simulink model "NCAP_AEBS_Test_T3_CCR_s_cs"  (Simulink 7.6)
settings: Solver=ode5  SolverMode=SingleTasking  StartTime=0.0  StopTime=inf  FixedStep=1/100  RelTol=1e-3
PreLoadFcn:
  | check_NUTS_defined;
  | 
  | assignin('base',['model_closed_' bdroot],false);addpath('../includes_AEBS');
InitFcn:
  | PreScanExperimentInitFcn(bdroot)
StopFcn:
  | PreScanExperimentStopFcn(bdroot)
undefined symbols (not defined in the file): DiscIntNeverNeededParam, x_ini_VRML, y_ini_VRML, z_ini_VRML
libraries: simulink x24, PreScanSimulinkLibrary x10, simulink_extras x7, PreScanUsefulBlocks x5, simulink_need_slupdate x1
(part 4 of 5)

== system NCAP_AEBS_Test_T3_CCR_s_cs/Audi_A8_1/PathFollower_1/CTRL REFERENCES ==
  note: REFERENCE POSITION BASED POSITION CTRL
  Pos x,y,Y [m,m,rad] : Inport
  Position Preview Distance [m] : Inport  Port=2
  TrajOffset [m,m,rad] : Inport  Port=3
  ActorOffset_Left(+) / Right(-)_[m] : Inport  Port=4
  Calculate Preview Point (pvp) by extrapolating current Vehicle Position (p0) with Preview Distance and Vehicle Orientation : Subsystem
  Find Reference Point (pref)  on Trajectory closest  to PreView Point (pvp) : M-S-Function  FunctionName=msfcn_find_closest_trajectory_points  Parameters=[Traj_x Traj_y]
      mask Display:
      | port_label('input', 1, 'pvp')
      | port_label('input', 2, 'TrajOffset_x_y_Y')
      | port_label('input', 3, 'ActorOffset_Left+/Right-')
      | port_label('input', 4, 'p0')
      | port_label('output', 1, 'pref')
  Find Reference Point (pref0)  on Trajectory closest  to P0 Point (p0) : M-S-Function  FunctionName=msfcn_find_closest_trajectory_points0  Parameters=[Traj_x Traj_y]
      mask Display:
      | port_label('input', 1, 'pvp')
      | port_label('input', 2, 'TrajOffset_x_y_Y')
      | port_label('input', 3, 'ActorOffset_Left+/Right-')
      | port_label('input', 4, 'p0')
      | port_label('output', 1, 'pref_0')
      | port_label('output', 2, 'Actor/Traj_distance')
      | port_label('output', 3, 'Actor/Traj_angle')
  Mux1 : Mux  Inputs=2
  Selector1 : Selector  InputPortWidth=3  IndexOptions=Index vector (dialog)  Indices=[1 2]  OutputSizes=1
  Terminator : Terminator
  pvp  [m,m] : Outport
  pref_pvp [m,m] : Outport  Port=2
  pref_0 [m,m] : Outport  Port=3
  Actor/Traj_distance [m] : Outport  Port=4
  Actor/Traj_angle [deg] : Outport  Port=5
  wires:
  Mux1/1 -> pvp  [m,m]/1, Find Reference Point (pref)  on Trajectory closest  to PreView Point (pvp)/1, Find Reference Point (pref0)  on Trajectory closest  to P0 Point (p0)/1
  Pos x,y,Y [m,m,rad]/1 -> Calculate Preview Point (pvp) by extrapolating current Vehicle Position (p0) with Preview Distance and Vehicle Orientation/2(x,y,Y Demux [m,m,rad]), Find Reference Point (pref0)  on Trajectory closest  to P0 Point (p0)/4, Selector1/1
  Calculate Preview Point (pvp) by extrapolating current Vehicle Position (p0) with Preview Distance and Vehicle Orientation/1(x_glob_PVD) -> Mux1/1
  Calculate Preview Point (pvp) by extrapolating current Vehicle Position (p0) with Preview Distance and Vehicle Orientation/3(Y [rad]) -> Terminator/1
  Position Preview Distance [m]/1 -> Calculate Preview Point (pvp) by extrapolating current Vehicle Position (p0) with Preview Distance and Vehicle Orientation/1(Preview Distance)
  Find Reference Point (pref)  on Trajectory closest  to PreView Point (pvp)/1 -> pref_pvp [m,m]/1
  Find Reference Point (pref0)  on Trajectory closest  to P0 Point (p0)/1 -> pref_0 [m,m]/1
  Calculate Preview Point (pvp) by extrapolating current Vehicle Position (p0) with Preview Distance and Vehicle Orientation/2(y_glob_PVD) -> Mux1/2
  TrajOffset [m,m,rad]/1 -> Find Reference Point (pref)  on Trajectory closest  to PreView Point (pvp)/2, Find Reference Point (pref0)  on Trajectory closest  to P0 Point (p0)/2  "L6"
  ActorOffset_Left(+) / Right(-)_[m]/1 -> Find Reference Point (pref)  on Trajectory closest  to PreView Point (pvp)/3, Find Reference Point (pref0)  on Trajectory closest  to P0 Point (p0)/3
  Selector1/1 -> Find Reference Point (pref)  on Trajectory closest  to PreView Point (pvp)/4
  Find Reference Point (pref0)  on Trajectory closest  to P0 Point (p0)/2 -> Actor/Traj_distance [m]/1
  Find Reference Point (pref0)  on Trajectory closest  to P0 Point (p0)/3 -> Actor/Traj_angle [deg]/1

== system NCAP_AEBS_Test_T3_CCR_s_cs/Audi_A8_1/PathFollower_1/Calculate shifted p0 wrt COG ==
  position x,y,Y [m,m,deg] : Inport
  Constant1 : Constant  Value=XShifting_wrt_COG
  Degrees to Radians : simulink_extras/Transformations/Degrees to Radians  SystemSampleTime=-1
  Demux1 : Demux  Outputs=3
  Fcn : Fcn  Expr=u(2)*cos(u(1))
  Fcn1 : Fcn  Expr=u(2)*sin(u(1))
  Mux1 : Mux  Inputs=3
  Mux2 : Mux  Inputs=2
  Sum : Sum  Inputs=|++
  Sum1 : Sum  Inputs=|++
  position x,y,Y [m,m,rad] : Outport
  wires:
  Sum/1 -> Mux1/1
  Sum1/1 -> Mux1/2
  Demux1/1 -> Sum/1
  Demux1/3 -> Degrees to Radians/1
  Degrees to Radians/1 -> Mux2/1, Mux1/3
  Mux2/1 -> Fcn/1, Fcn1/1
  Fcn/1 -> Sum/2
  Fcn1/1 -> Sum1/2
  Demux1/2 -> Sum1/1
  position x,y,Y [m,m,deg]/1 -> Demux1/1
  Mux1/1 -> position x,y,Y [m,m,rad]/1
  Constant1/1 -> Mux2/2

== system NCAP_AEBS_Test_T3_CCR_s_cs/Audi_A8_1/PathFollower_1/DELTA CTRL ==
  note: POSITION BASED STEERWHEEL CONTROL
  p0 : Inport
  pvp : Inport  Port=2
  pref_pvp : Inport  Port=3
  pref0 : Inport  Port=4
  Calculate  preview angle : M-S-Function  FunctionName=msfcn_preview_angle_and_distance
      mask Display:
      | port_label('input', 2, 'pref [m,m]')
      | port_label('input', 3, 'p0 [m,m]')
      | port_label('input', 1, 'pvp [m,m]')
      | 
      | port_label('output', 1, 'angle [rad]')
  Divide2 : Product
  Divide4 : Product
  Error check : Subsystem
  Goto Tag Visibility : GotoTagVisibility  GotoTag=pref0
  Goto Tag Visibility1 : GotoTagVisibility  GotoTag=p0
  Radians to Degrees1 : simulink_extras/Transformations/Radians to Degrees  SystemSampleTime=-1
  Selector2 : Selector  InputPortWidth=3  IndexOptions=Index vector (dialog)  Indices=[1 2]  OutputSizes=1
  Steering angle  velocity dependent : Lookup  InputValues=[0 18 40 60 70 80 90 100 110]  Table=[16.5 16.5 28 44.5 55 60.5 60.5 60.5 60.5]
  Steering angle preview  distance dependent : Lookup  InputValues=[0 1 4 5 6 7 8 9 10 11 20 21]  Table=[1.5 1.5 1 1 1 1 1 1 0.9 0.9 0.8 0.8]
  These limits are  the vehicle maximum  steering wheel angle : Saturate  UpperLimit=720  LowerLimit=-720
  TunableSteering Gain : Gain  Gain=TunableSteeringGain
  sign1 : Gain  Gain=3.6
  delta_steerwheel [deg] : Outport
  tag scope: p0=scoped, pref0=scoped
  wires:
  Calculate  preview angle/1 -> Radians to Degrees1/1
  Selector2/1 -> Calculate  preview angle/3
  p0/1 -> Selector2/1, [p0]
  pvp/1 -> Calculate  preview angle/1
  pref_pvp/1 -> Calculate  preview angle/2
  Radians to Degrees1/1 -> Divide2/2
  These limits are  the vehicle maximum  steering wheel angle/1 -> delta_steerwheel [deg]/1
  pref0/1 -> [pref0]
  sign1/1 -> Steering angle  velocity dependent/1
  [v_actual] -> sign1/1
  Steering angle  velocity dependent/1 -> Divide2/1
  Divide4/1 -> TunableSteering Gain/1
  Divide2/1 -> Divide4/1
  Steering angle preview  distance dependent/1 -> Divide4/2
  [PreviewDistance] -> Steering angle preview  distance dependent/1
  TunableSteering Gain/1 -> These limits are  the vehicle maximum  steering wheel angle/1

== system NCAP_AEBS_Test_T3_CCR_s_cs/Audi_A8_1/PathFollower_1/THROTTLE CTRL ==
  v_actual [m/s] : Inport
  Desired Velocity [m/s] : Inport  Port=2
  Initial Velocity [m/s] : Inport  Port=3
  Demux : Demux  Outputs=3
  GearNormal : Constant
  "GearNormal " : Constant
  If Desired Velocity = 0 : Subsystem  TreatAsAtomicUnit=on
  If Desired Velocity ~= 0 : Subsystem  TreatAsAtomicUnit=on
  Merge : Merge
  Mux : Mux  Inputs=3
  Mux2 : Mux  Inputs=3
  Sum4 : Sum  Inputs=|+-
  if : If  IfExpression=u1 == 0
  throttle [%] : Outport
  brake pressure [bar] : Outport  Port=2
  v0 [m/s] : Outport  Port=3
  Auto_GearShift : Outport  Port=4
  wires:
  v_actual [m/s]/1 -> Sum4/2
  If Desired Velocity ~= 0/3(Auto_GearShift) -> Mux2/3
  If Desired Velocity ~= 0/2(brake pressure [bar]) -> Mux2/2
  If Desired Velocity ~= 0/1(throttle [%]) -> Mux2/1
  if/1 -> If Desired Velocity = 0/Action
  if/2 -> If Desired Velocity ~= 0/Action
  If Desired Velocity = 0/3(Auto_GearShift) -> Mux/3
  "GearNormal "/1 -> If Desired Velocity ~= 0/1(In1)
  Demux/3 -> Auto_GearShift/1
  Demux/2 -> brake pressure [bar]/1
  Demux/1 -> throttle [%]/1
  Mux/1 -> Merge/1
  Mux2/1 -> Merge/2
  If Desired Velocity = 0/2(brake pressure [bar]) -> Mux/2
  If Desired Velocity = 0/1(throttle [%]) -> Mux/1
  Merge/1 -> Demux/1
  GearNormal/1 -> If Desired Velocity = 0/1(In1)
  Initial Velocity [m/s]/1 -> v0 [m/s]/1
  Desired Velocity [m/s]/1 -> Sum4/1, if/1
  Sum4/1 -> If Desired Velocity ~= 0/2(Desired Velocity [m/s])

== system NCAP_AEBS_Test_T3_CCR_s_cs/Audi_A8_1/SELF_Demux/compas converter ==
  rotz [rad] : Inport
  cart2compas : Subsystem
  rad2deg : Gain  Gain=180/pi
  heading [deg] : Outport
  wires:
  cart2compas/1(heading [deg]) -> heading [deg]/1
  rotz [rad]/1 -> rad2deg/1
  rad2deg/1 -> cart2compas/1(Angle [deg])

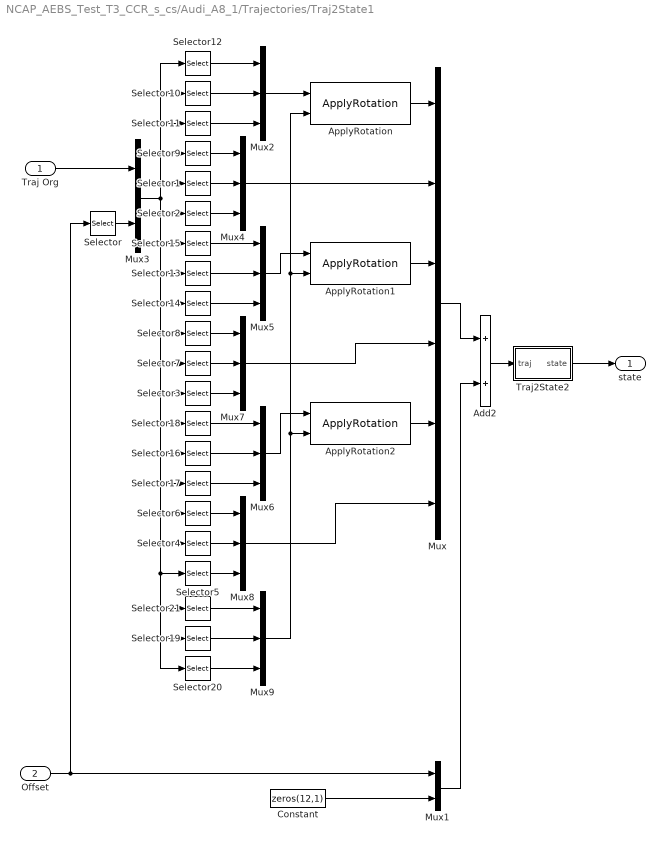
== system NCAP_AEBS_Test_T3_CCR_s_cs/Audi_A8_1/Trajectories/Traj2State1 ==
  Traj Org : Inport
  Offset : Inport  Port=2
  Add2 : Sum
  ApplyRotation : PreScanSimulinkLibrary/ApplyRotation  SystemSampleTime=-1
  ApplyRotation1 : PreScanSimulinkLibrary/ApplyRotation  SystemSampleTime=-1
  ApplyRotation2 : PreScanSimulinkLibrary/ApplyRotation  SystemSampleTime=-1
  Constant : Constant  Value=zeros(12,1)
  Mux : Mux  Inputs=6
  Mux1 : Mux  Inputs=2
  Mux{2,4..9} (7 alike) : Mux  Inputs=3
  Mux3 : Mux  Inputs=2
  Selector : Selector  InputPortWidth=6  IndexOptions=Index vector (dialog)  Indices=[4 5 6]  OutputSizes=1
  Selector1 : Selector  InputPortWidth=21  IndexOptions=Index vector (dialog)  Indices=[5]  OutputSizes=1
  Selector10 : Selector  InputPortWidth=21  IndexOptions=Index vector (dialog)  Indices=[2]  OutputSizes=1
  Selector11 : Selector  InputPortWidth=21  IndexOptions=Index vector (dialog)  Indices=[3]  OutputSizes=1
  Selector12 : Selector  InputPortWidth=21  IndexOptions=Index vector (dialog)  Indices=[1]  OutputSizes=1
  Selector13 : Selector  InputPortWidth=21  IndexOptions=Index vector (dialog)  Indices=[8]  OutputSizes=1
  Selector14 : Selector  InputPortWidth=21  IndexOptions=Index vector (dialog)  Indices=[9]  OutputSizes=1
  Selector15 : Selector  InputPortWidth=21  IndexOptions=Index vector (dialog)  Indices=[7]  OutputSizes=1
  Selector16 : Selector  InputPortWidth=21  IndexOptions=Index vector (dialog)  Indices=[14]  OutputSizes=1
  Selector17 : Selector  InputPortWidth=21  IndexOptions=Index vector (dialog)  Indices=[15]  OutputSizes=1
  Selector18 : Selector  InputPortWidth=21  IndexOptions=Index vector (dialog)  Indices=[13]  OutputSizes=1
  Selector19 : Selector  InputPortWidth=21  IndexOptions=Index vector (dialog)  Indices=[20]  OutputSizes=1
  Selector2 : Selector  InputPortWidth=21  IndexOptions=Index vector (dialog)  Indices=[6]  OutputSizes=1
  Selector20 : Selector  InputPortWidth=21  IndexOptions=Index vector (dialog)  Indices=[21]  OutputSizes=1
  Selector21 : Selector  InputPortWidth=21  IndexOptions=Index vector (dialog)  Indices=[19]  OutputSizes=1
  Selector3 : Selector  InputPortWidth=21  IndexOptions=Index vector (dialog)  Indices=[12]  OutputSizes=1
  Selector4 : Selector  InputPortWidth=21  IndexOptions=Index vector (dialog)  Indices=[17]  OutputSizes=1
  Selector5 : Selector  InputPortWidth=21  IndexOptions=Index vector (dialog)  Indices=[18]  OutputSizes=1
  Selector6 : Selector  InputPortWidth=21  IndexOptions=Index vector (dialog)  Indices=[16]  OutputSizes=1
  Selector7 : Selector  InputPortWidth=21  IndexOptions=Index vector (dialog)  Indices=[11]  OutputSizes=1
  Selector8 : Selector  InputPortWidth=21  IndexOptions=Index vector (dialog)  Indices=[10]  OutputSizes=1
  Selector9 : Selector  InputPortWidth=21  IndexOptions=Index vector (dialog)  Indices=[4]  OutputSizes=1
  Traj2State2 : Subsystem
  state : Outport
  wires:
  Mux9/1 -> ApplyRotation2/2, ApplyRotation1/2, ApplyRotation/2
  Selector20/1 -> Mux9/3
  Selector19/1 -> Mux9/2
  Selector21/1 -> Mux9/1
  Selector5/1 -> Mux8/3
  Selector4/1 -> Mux8/2
  Selector6/1 -> Mux8/1
  Mux8/1 -> Mux/6
  Mux6/1 -> ApplyRotation2/1
  Mux7/1 -> Mux/4
  ApplyRotation2/1 -> Mux/5
  Selector3/1 -> Mux7/3
  Selector7/1 -> Mux7/2
  Selector8/1 -> Mux7/1
  Mux4/1 -> Mux/2
  Mux5/1 -> ApplyRotation1/1
  ApplyRotation1/1 -> Mux/3
  Mux2/1 -> ApplyRotation/1
  ApplyRotation/1 -> Mux/1
  Selector2/1 -> Mux4/3
  Selector1/1 -> Mux4/2
  Selector9/1 -> Mux4/1
  Selector17/1 -> Mux6/3
  Selector16/1 -> Mux6/2
  Selector18/1 -> Mux6/1
  Selector14/1 -> Mux5/3
  Selector13/1 -> Mux5/2
  Selector15/1 -> Mux5/1
  Selector11/1 -> Mux2/3
  Selector10/1 -> Mux2/2
  Selector12/1 -> Mux2/1
  Mux3/1 -> Selector8/1, Selector7/1, Selector3/1, Selector18/1, Selector16/1, Selector17/1, Selector6/1, Selector20/1, Selector19/1, Selector21/1, Selector5/1, Selector4/1, Selector14/1, Selector13/1, Selector15/1, Selector2/1, Selector1/1, Selector9/1, Selector12/1, Selector10/1, Selector11/1
  Mux1/1 -> Add2/2
  Constant/1 -> Mux1/2
  Add2/1 -> Traj2State2/1(traj)
  Selector/1 -> Mux3/2
  Traj Org/1 -> Mux3/1
  Offset/1 -> Mux1/1, Selector/1
  Mux/1 -> Add2/1
  Traj2State2/1(state) -> state/1

== system NCAP_AEBS_Test_T3_CCR_s_cs/Audi_A8_1/Trajectories/Trajectory_1 ==
  From Workspace : FromWorkspace  VariableName=trajectory  SampleTime=TimeStep  OutputAfterFinalValue=Holding final value
  From Workspace1 : FromWorkspace  VariableName=trajectory  SampleTime=TimeStep  OutputAfterFinalValue=Setting to zero
  Mux : Mux  Inputs=2
  Selector1 : Selector  InputPortWidth=24  IndexOptions=Index vector (dialog)  Indices=[7:18]  OutputSizes=1
  Selector9 : Selector  InputPortWidth=24  IndexOptions=Index vector (dialog)  Indices=[1:6]  OutputSizes=1
  trajectory : Outport
  wires:
  Selector1/1 -> Mux/2
  Selector9/1 -> Mux/1
  Mux/1 -> trajectory/1
  From Workspace1/1 -> Selector1/1
  From Workspace/1 -> Selector9/1

== system NCAP_AEBS_Test_T3_CCR_s_cs/BalloonCar_1/Dynamics_Empty/MuxState ==
  note: mode: Dynamics
  note: mode: Positioning
  note: mode: Dynamics
      | VelVEHICLE
      | wrt VEH
  note: AnglesVEHICLE
      | wrtGLOB
  note: For state mode 'Dynamic' positions
      | are not taken into account, as they
      | are computed by integrating velocity.
      | Click annotation for Help.
  x [m] : Inport  SampleTime=TimeStep
  y [m] : Inport  Port=2  SampleTime=TimeStep
  z [m] : Inport  Port=3  SampleTime=TimeStep
  dx [m/s] : Inport  Port=4  SampleTime=TimeStep
  dy [m/s] : Inport  Port=5  SampleTime=TimeStep
  dz [m/s] : Inport  Port=6  SampleTime=TimeStep
  R [rad] : Inport  Port=7  SampleTime=TimeStep
  P [rad] : Inport  Port=8  SampleTime=TimeStep
  Y [rad] : Inport  Port=9  SampleTime=TimeStep
  Constant : Constant  DisableCoverage=on  Value=positioningmode
  Discrete-Time Integrator : DiscreteIntegrator  SampleTime=TimeStep  ICPrevOutput=DiscIntNeverNeededParam  ICPrevScaledInput=DiscIntNeverNeededParam
  Ground : Ground
  Ground1 : Ground
  Mux1 : Mux  Inputs=[3 3]
  Mux2 : Mux  Inputs=3
  Mux3 : Mux  Inputs=3
  Mux4 : Mux  Inputs=3
  Mux5 : Mux  Inputs=[3 3]
  Mux6 : Mux  Inputs=[6 3]
  Switch : Switch  Threshold=0.5
  Transformation_BODY2GLOBAL : PreScanSimulinkLibrary/Simple_Vehicle_Dynamics/Chassis/MuxDynState/Transformation_BODY2GLOBAL  SystemSampleTime=-1
  mux3 : Mux  Inputs=3
  state : Outport
  wires:
  Constant/1 -> Switch/2
  Mux6/1 -> state/1
  Mux4/1 -> Mux1/1
  Mux5/1 -> Switch/3
  Mux1/1 -> Switch/1
  Switch/1 -> Mux6/1  "PosVeh wrt  GLOB"
  P [rad]/1 -> Mux3/2
  R [rad]/1 -> Mux3/1
  dz [m/s]/1 -> Mux2/3
  dy [m/s]/1 -> Mux2/2
  dx [m/s]/1 -> Mux2/1
  z [m]/1 -> Mux4/3
  y [m]/1 -> Mux4/2
  x [m]/1 -> Mux4/1
  Ground1/1 -> mux3/2  "pitch"
  Y [rad]/1 -> mux3/3, Mux3/3  "yaw"
  Mux3/1 -> Mux6/2
  Transformation_BODY2GLOBAL/1 -> Discrete-Time Integrator/1, Mux5/2  "VelVEH wrt  GLOB"
  mux3/1 -> Transformation_BODY2GLOBAL/2
  Ground/1 -> mux3/1  "roll"
  Mux2/1 -> Mux1/2, Transformation_BODY2GLOBAL/1
  Discrete-Time Integrator/1 -> Mux5/1  "PosVEH wrt  GLOB"

== system NCAP_AEBS_Test_T3_CCR_s_cs/BalloonCar_1/SELF_Demux/compas converter ==
  rotz [rad] : Inport
  cart2compas : Subsystem
  rad2deg : Gain  Gain=180/pi
  heading [deg] : Outport
  wires:
  cart2compas/1(heading [deg]) -> heading [deg]/1
  rotz [rad]/1 -> rad2deg/1
  rad2deg/1 -> cart2compas/1(Angle [deg])

== system NCAP_AEBS_Test_T3_CCR_s_cs/Sphere_1/Dynamics_Empty/MuxState ==
  note: mode: Dynamics
  note: mode: Positioning
  note: mode: Dynamics
      | VelVEHICLE
      | wrt VEH
  note: AnglesVEHICLE
      | wrtGLOB
  note: For state mode 'Dynamic' positions
      | are not taken into account, as they
      | are computed by integrating velocity.
      | Click annotation for Help.
  x [m] : Inport  SampleTime=TimeStep
  y [m] : Inport  Port=2  SampleTime=TimeStep
  z [m] : Inport  Port=3  SampleTime=TimeStep
  dx [m/s] : Inport  Port=4  SampleTime=TimeStep
  dy [m/s] : Inport  Port=5  SampleTime=TimeStep
  dz [m/s] : Inport  Port=6  SampleTime=TimeStep
  R [rad] : Inport  Port=7  SampleTime=TimeStep
  P [rad] : Inport  Port=8  SampleTime=TimeStep
  Y [rad] : Inport  Port=9  SampleTime=TimeStep
  Constant : Constant  DisableCoverage=on  Value=positioningmode
  Discrete-Time Integrator : DiscreteIntegrator  SampleTime=TimeStep  ICPrevOutput=DiscIntNeverNeededParam  ICPrevScaledInput=DiscIntNeverNeededParam
  Ground : Ground
  Ground1 : Ground
  Mux1 : Mux  Inputs=[3 3]
  Mux2 : Mux  Inputs=3
  Mux3 : Mux  Inputs=3
  Mux4 : Mux  Inputs=3
  Mux5 : Mux  Inputs=[3 3]
  Mux6 : Mux  Inputs=[6 3]
  Switch : Switch  Threshold=0.5
  Transformation_BODY2GLOBAL : PreScanSimulinkLibrary/Simple_Vehicle_Dynamics/Chassis/MuxDynState/Transformation_BODY2GLOBAL  SystemSampleTime=-1
  mux3 : Mux  Inputs=3
  state : Outport
  wires:
  Constant/1 -> Switch/2
  Mux6/1 -> state/1
  Mux4/1 -> Mux1/1
  Mux5/1 -> Switch/3
  Mux1/1 -> Switch/1
  Switch/1 -> Mux6/1  "PosVeh wrt  GLOB"
  P [rad]/1 -> Mux3/2
  R [rad]/1 -> Mux3/1
  dz [m/s]/1 -> Mux2/3
  dy [m/s]/1 -> Mux2/2
  dx [m/s]/1 -> Mux2/1
  z [m]/1 -> Mux4/3
  y [m]/1 -> Mux4/2
  x [m]/1 -> Mux4/1
  Ground1/1 -> mux3/2  "pitch"
  Y [rad]/1 -> mux3/3, Mux3/3  "yaw"
  Mux3/1 -> Mux6/2
  Transformation_BODY2GLOBAL/1 -> Discrete-Time Integrator/1, Mux5/2  "VelVEH wrt  GLOB"
  mux3/1 -> Transformation_BODY2GLOBAL/2
  Ground/1 -> mux3/1  "roll"
  Mux2/1 -> Mux1/2, Transformation_BODY2GLOBAL/1
  Discrete-Time Integrator/1 -> Mux5/1  "PosVEH wrt  GLOB"

== system NCAP_AEBS_Test_T3_CCR_s_cs/Sphere_1/SELF_Demux/compas converter ==
  rotz [rad] : Inport
  cart2compas : Subsystem
  rad2deg : Gain  Gain=180/pi
  heading [deg] : Outport
  wires:
  cart2compas/1(heading [deg]) -> heading [deg]/1
  rotz [rad]/1 -> rad2deg/1
  rad2deg/1 -> cart2compas/1(Angle [deg])

== system NCAP_AEBS_Test_T3_CCR_s_cs/VISUWheels_Audi_A8_1/conv_RotWheelFL/RotMat2AxisAngle ==
  RotMat_Visu : Inport
  Data Type Conversion : DataTypeConversion
  Divide : Product  Inputs=*/
  Gain : Gain  Gain=2
  Mux : Mux  Inputs=3
  Mux1 : Mux  Inputs=2
  Saturation1 : Saturate  UpperLimit=3-0.001  LowerLimit=-1+0.001
  Trigonometric Function : Trigonometry
  U1 : Fcn  Expr=u[6]-u[8]
  U2 : Fcn  Expr=u[7]-u[3]
  U3 : Fcn  Expr=u[2]-u[4]
  U_Phi : Fcn  Expr=u[1]+u[5]+u[9]
  U_Phi1 : Fcn  Expr=acos((u(1)-1)/2)
  U_Phi2 : Fcn  Expr=acos((u(1)-1)/2)
  Angles_Visu : Outport
  wires:
  U_Phi2/1 -> Trigonometric Function/1
  Saturation1/1 -> U_Phi2/1
  U_Phi1/1 -> Data Type Conversion/1
  U_Phi/1 -> Saturation1/1, U_Phi1/1
  Divide/1 -> Mux1/1
  Mux1/1 -> Angles_Visu/1
  Gain/1 -> Divide/2
  Mux/1 -> Divide/1
  U3/1 -> Mux/3
  U2/1 -> Mux/2
  U1/1 -> Mux/1
  Trigonometric Function/1 -> Gain/1
  RotMat_Visu/1 -> U_Phi/1, U3/1, U2/1, U1/1
  Data Type Conversion/1 -> Mux1/2

== system NCAP_AEBS_Test_T3_CCR_s_cs/VISUWheels_Audi_A8_1/conv_RotWheelFR/RotMat2AxisAngle ==
  RotMat_Visu : Inport
  Data Type Conversion : DataTypeConversion
  Divide : Product  Inputs=*/
  Gain : Gain  Gain=2
  Mux : Mux  Inputs=3
  Mux1 : Mux  Inputs=2
  Saturation1 : Saturate  UpperLimit=3-0.001  LowerLimit=-1+0.001
  Trigonometric Function : Trigonometry
  U1 : Fcn  Expr=u[6]-u[8]
  U2 : Fcn  Expr=u[7]-u[3]
  U3 : Fcn  Expr=u[2]-u[4]
  U_Phi : Fcn  Expr=u[1]+u[5]+u[9]
  U_Phi1 : Fcn  Expr=acos((u(1)-1)/2)
  U_Phi2 : Fcn  Expr=acos((u(1)-1)/2)
  Angles_Visu : Outport
  wires:
  Data Type Conversion/1 -> Mux1/2
  RotMat_Visu/1 -> U1/1, U2/1, U3/1, U_Phi/1
  Trigonometric Function/1 -> Gain/1
  U1/1 -> Mux/1
  U2/1 -> Mux/2
  U3/1 -> Mux/3
  Mux/1 -> Divide/1
  Gain/1 -> Divide/2
  Mux1/1 -> Angles_Visu/1
  Divide/1 -> Mux1/1
  U_Phi/1 -> U_Phi1/1, Saturation1/1
  U_Phi1/1 -> Data Type Conversion/1
  Saturation1/1 -> U_Phi2/1
  U_Phi2/1 -> Trigonometric Function/1

== system NCAP_AEBS_Test_T3_CCR_s_cs/VISUWheels_Audi_A8_1/conv_RotWheelRL/RotMat2AxisAngle ==
  RotMat_Visu : Inport
  Data Type Conversion : DataTypeConversion
  Divide : Product  Inputs=*/
  Gain : Gain  Gain=2
  Mux : Mux  Inputs=3
  Mux1 : Mux  Inputs=2
  Saturation1 : Saturate  UpperLimit=3-0.001  LowerLimit=-1+0.001
  Trigonometric Function : Trigonometry
  U1 : Fcn  Expr=u[6]-u[8]
  U2 : Fcn  Expr=u[7]-u[3]
  U3 : Fcn  Expr=u[2]-u[4]
  U_Phi : Fcn  Expr=u[1]+u[5]+u[9]
  U_Phi1 : Fcn  Expr=acos((u(1)-1)/2)
  U_Phi2 : Fcn  Expr=acos((u(1)-1)/2)
  Angles_Visu : Outport
  wires:
  Data Type Conversion/1 -> Mux1/2
  RotMat_Visu/1 -> U1/1, U2/1, U3/1, U_Phi/1
  Trigonometric Function/1 -> Gain/1
  U1/1 -> Mux/1
  U2/1 -> Mux/2
  U3/1 -> Mux/3
  Mux/1 -> Divide/1
  Gain/1 -> Divide/2
  Mux1/1 -> Angles_Visu/1
  Divide/1 -> Mux1/1
  U_Phi/1 -> U_Phi1/1, Saturation1/1
  U_Phi1/1 -> Data Type Conversion/1
  Saturation1/1 -> U_Phi2/1
  U_Phi2/1 -> Trigonometric Function/1

== system NCAP_AEBS_Test_T3_CCR_s_cs/VISUWheels_Audi_A8_1/conv_RotWheelRR/RotMat2AxisAngle ==
  RotMat_Visu : Inport
  Data Type Conversion : DataTypeConversion
  Divide : Product  Inputs=*/
  Gain : Gain  Gain=2
  Mux : Mux  Inputs=3
  Mux1 : Mux  Inputs=2
  Saturation1 : Saturate  UpperLimit=3-0.001  LowerLimit=-1+0.001
  Trigonometric Function : Trigonometry
  U1 : Fcn  Expr=u[6]-u[8]
  U2 : Fcn  Expr=u[7]-u[3]
  U3 : Fcn  Expr=u[2]-u[4]
  U_Phi : Fcn  Expr=u[1]+u[5]+u[9]
  U_Phi1 : Fcn  Expr=acos((u(1)-1)/2)
  U_Phi2 : Fcn  Expr=acos((u(1)-1)/2)
  Angles_Visu : Outport
  wires:
  Data Type Conversion/1 -> Mux1/2
  RotMat_Visu/1 -> U1/1, U2/1, U3/1, U_Phi/1
  Trigonometric Function/1 -> Gain/1
  U1/1 -> Mux/1
  U2/1 -> Mux/2
  U3/1 -> Mux/3
  Mux/1 -> Divide/1
  Gain/1 -> Divide/2
  Mux1/1 -> Angles_Visu/1
  Divide/1 -> Mux1/1
  U_Phi/1 -> U_Phi1/1, Saturation1/1
  U_Phi1/1 -> Data Type Conversion/1
  Saturation1/1 -> U_Phi2/1
  U_Phi2/1 -> Trigonometric Function/1

== system NCAP_AEBS_Test_T3_CCR_s_cs/VISUWheels_Audi_A8_1/conv_TransWheelFL/pos_ini_Visu ==
  Constant : Constant  Value=x_ini_VRML
  Constant1 : Constant  Value=y_ini_VRML
  Constant2 : Constant  Value=z_ini_VRML
  Mux1 : Mux  Inputs=3
  pos_ini_Visu : Outport
  wires:
  Constant2/1 -> Mux1/3
  Constant1/1 -> Mux1/2
  Mux1/1 -> pos_ini_Visu/1
  Constant/1 -> Mux1/1

== system NCAP_AEBS_Test_T3_CCR_s_cs/VISUWheels_Audi_A8_1/conv_TransWheelFL/transISO2Visu ==
  transISO : Inport
  Demux : Demux  Outputs=3
  trans_x_Visu : Outport
  trans_y_Visu : Outport  Port=2
  trans_z_Visu : Outport  Port=3
  wires:
  Demux/3 -> trans_z_Visu/1
  transISO/1 -> Demux/1
  Demux/1 -> trans_x_Visu/1
  Demux/2 -> trans_y_Visu/1  "rot_y"

== system NCAP_AEBS_Test_T3_CCR_s_cs/VISUWheels_Audi_A8_1/conv_TransWheelFR/pos_ini_Visu ==
  Constant : Constant  Value=x_ini_VRML
  Constant1 : Constant  Value=y_ini_VRML
  Constant2 : Constant  Value=z_ini_VRML
  Mux1 : Mux  Inputs=3
  pos_ini_Visu : Outport
  wires:
  Constant/1 -> Mux1/1
  Mux1/1 -> pos_ini_Visu/1
  Constant1/1 -> Mux1/2
  Constant2/1 -> Mux1/3

== system NCAP_AEBS_Test_T3_CCR_s_cs/VISUWheels_Audi_A8_1/conv_TransWheelFR/transISO2Visu ==
  transISO : Inport
  Demux : Demux  Outputs=3
  trans_x_Visu : Outport
  trans_y_Visu : Outport  Port=2
  trans_z_Visu : Outport  Port=3
  wires:
  Demux/3 -> trans_z_Visu/1
  transISO/1 -> Demux/1
  Demux/1 -> trans_x_Visu/1
  Demux/2 -> trans_y_Visu/1  "rot_y"

== system NCAP_AEBS_Test_T3_CCR_s_cs/VISUWheels_Audi_A8_1/conv_TransWheelRL/pos_ini_Visu ==
  Constant : Constant  Value=x_ini_VRML
  Constant1 : Constant  Value=y_ini_VRML
  Constant2 : Constant  Value=z_ini_VRML
  Mux1 : Mux  Inputs=3
  pos_ini_Visu : Outport
  wires:
  Constant/1 -> Mux1/1
  Mux1/1 -> pos_ini_Visu/1
  Constant1/1 -> Mux1/2
  Constant2/1 -> Mux1/3

== system NCAP_AEBS_Test_T3_CCR_s_cs/VISUWheels_Audi_A8_1/conv_TransWheelRL/transISO2Visu ==
  transISO : Inport
  Demux : Demux  Outputs=3
  trans_x_Visu : Outport
  trans_y_Visu : Outport  Port=2
  trans_z_Visu : Outport  Port=3
  wires:
  Demux/3 -> trans_z_Visu/1
  transISO/1 -> Demux/1
  Demux/1 -> trans_x_Visu/1
  Demux/2 -> trans_y_Visu/1  "rot_y"

== system NCAP_AEBS_Test_T3_CCR_s_cs/VISUWheels_Audi_A8_1/conv_TransWheelRR/pos_ini_Visu ==
  Constant : Constant  Value=x_ini_VRML
  Constant1 : Constant  Value=y_ini_VRML
  Constant2 : Constant  Value=z_ini_VRML
  Mux1 : Mux  Inputs=3
  pos_ini_Visu : Outport
  wires:
  Constant/1 -> Mux1/1
  Mux1/1 -> pos_ini_Visu/1
  Constant1/1 -> Mux1/2
  Constant2/1 -> Mux1/3

== system NCAP_AEBS_Test_T3_CCR_s_cs/VISUWheels_Audi_A8_1/conv_TransWheelRR/transISO2Visu ==
  transISO : Inport
  Demux : Demux  Outputs=3
  trans_x_Visu : Outport
  trans_y_Visu : Outport  Port=2
  trans_z_Visu : Outport  Port=3
  wires:
  Demux/3 -> trans_z_Visu/1
  transISO/1 -> Demux/1
  Demux/1 -> trans_x_Visu/1
  Demux/2 -> trans_y_Visu/1  "rot_y"

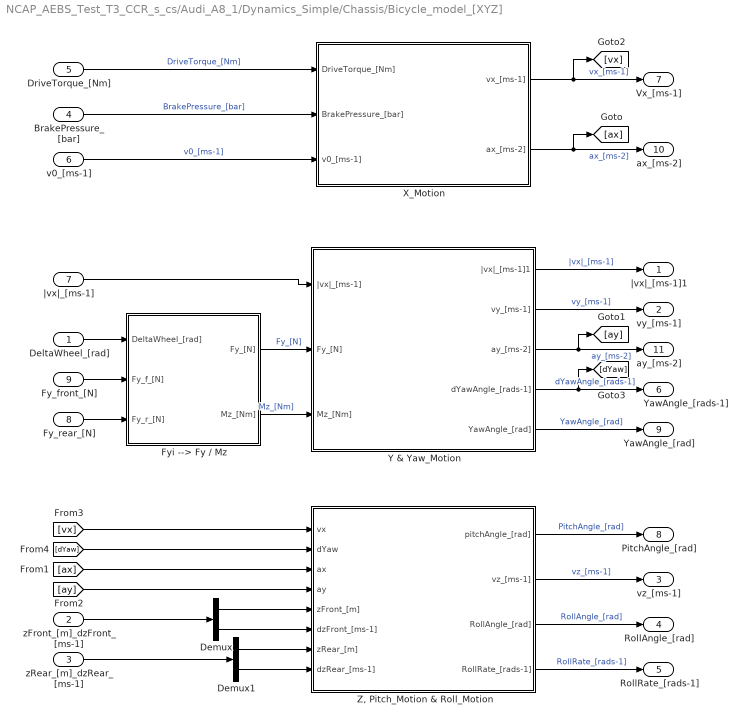
== system NCAP_AEBS_Test_T3_CCR_s_cs/Audi_A8_1/Dynamics_Simple/Chassis/Bicycle_model_[XYZ] ==
  DeltaWheel_[rad] : Inport
  zFront_[m]_dzFront_[ms-1] : Inport  Port=2  PortDimensions=2
  zRear_[m]_dzRear_[ms-1] : Inport  Port=3  PortDimensions=2
  BrakePressure_[bar] : Inport  Port=4
  DriveTorque_[Nm] : Inport  Port=5
  v0_[ms-1] : Inport  Port=6
  |vx|_[ms-1] : Inport  Port=7
  Fy_rear_[N] : Inport  Port=8
  Fy_front_[N] : Inport  Port=9
  Demux : Demux  Outputs=2
  Demux1 : Demux  Outputs=2
  Fyi --> Fy / Mz : Subsystem
  X_Motion : Subsystem
  Y & Yaw_Motion : Subsystem
  "Z, Pitch_Motion & Roll_Motion" : Subsystem
  |vx|_[ms-1]1 : Outport
  vy_[ms-1] : Outport  Port=2
  vz_[ms-1] : Outport  Port=3
  RollAngle_[rad] : Outport  Port=4
  RollRate_[rads-1] : Outport  Port=5
  YawAngle_[rads-1] : Outport  Port=6
  Vx_[ms-1] : Outport  Port=7
  PitchAngle_[rad] : Outport  Port=8
  YawAngle_[rad] : Outport  Port=9
  ax_[ms-2] : Outport  Port=10
  ay_[ms-2] : Outport  Port=11
  wires:
  Fyi --> Fy / Mz/1(Fy_[N]) -> Y & Yaw_Motion/2(Fy_[N])  "Fy_[N]"
  Fyi --> Fy / Mz/2(Mz_[Nm]) -> Y & Yaw_Motion/3(Mz_[Nm])  "Mz_[Nm]"
  Y & Yaw_Motion/1(|vx|_[ms-1]1) -> |vx|_[ms-1]1/1  "|vx|_[ms-1]"
  Y & Yaw_Motion/2(vy_[ms-1]) -> vy_[ms-1]/1  "vy_[ms-1]"
  Y & Yaw_Motion/5(YawAngle_[rad]) -> YawAngle_[rad]/1  "YawAngle_[rad]"
  v0_[ms-1]/1 -> X_Motion/3(v0_[ms-1])  "v0_[ms-1]"
  BrakePressure_[bar]/1 -> X_Motion/2(BrakePressure_[bar])  "BrakePressure_[bar]"
  DriveTorque_[Nm]/1 -> X_Motion/1(DriveTorque_[Nm])  "DriveTorque_[Nm]"
  X_Motion/2(ax_[ms-2]) -> ax_[ms-2]/1, [ax]  "ax_[ms-2]"
  X_Motion/1(vx_[ms-1]) -> Vx_[ms-1]/1, [vx]  "vx_[ms-1]"
  [ax] -> "Z, Pitch_Motion & Roll_Motion"/3(ax)
  Demux/1 -> "Z, Pitch_Motion & Roll_Motion"/5(zFront_[m])
  Demux/2 -> "Z, Pitch_Motion & Roll_Motion"/6(dzFront_[ms-1])
  Demux1/1 -> "Z, Pitch_Motion & Roll_Motion"/7(zRear_[m])
  Demux1/2 -> "Z, Pitch_Motion & Roll_Motion"/8(dzRear_[ms-1])
  zRear_[m]_dzRear_[ms-1]/1 -> Demux1/1
  zFront_[m]_dzFront_[ms-1]/1 -> Demux/1
  "Z, Pitch_Motion & Roll_Motion"/2(vz_[ms-1]) -> vz_[ms-1]/1  "vz_[ms-1]"
  DeltaWheel_[rad]/1 -> Fyi --> Fy / Mz/1(DeltaWheel_[rad])
  Fy_front_[N]/1 -> Fyi --> Fy / Mz/2(Fy_f_[N])
  Fy_rear_[N]/1 -> Fyi --> Fy / Mz/3(Fy_r_[N])
  |vx|_[ms-1]/1 -> Y & Yaw_Motion/1(|vx|_[ms-1])
  Y & Yaw_Motion/3(ay_[ms-2]) -> [ay], ay_[ms-2]/1  "ay_[ms-2]"
  [ay] -> "Z, Pitch_Motion & Roll_Motion"/4(ay)
  "Z, Pitch_Motion & Roll_Motion"/3(RollAngle_[rad]) -> RollAngle_[rad]/1  "RollAngle_[rad]"
  "Z, Pitch_Motion & Roll_Motion"/4(RollRate_[rads-1]) -> RollRate_[rads-1]/1  "RollRate_[rads-1]"
  [dYaw] -> "Z, Pitch_Motion & Roll_Motion"/2(dYaw)
  [vx] -> "Z, Pitch_Motion & Roll_Motion"/1(vx)
  Y & Yaw_Motion/4(dYawAngle_[rads-1]) -> YawAngle_[rads-1]/1, [dYaw]  "dYawAngle_[rads-1]"
  "Z, Pitch_Motion & Roll_Motion"/1(pitchAngle_[rad]) -> PitchAngle_[rad]/1  "PitchAngle_[rad]"

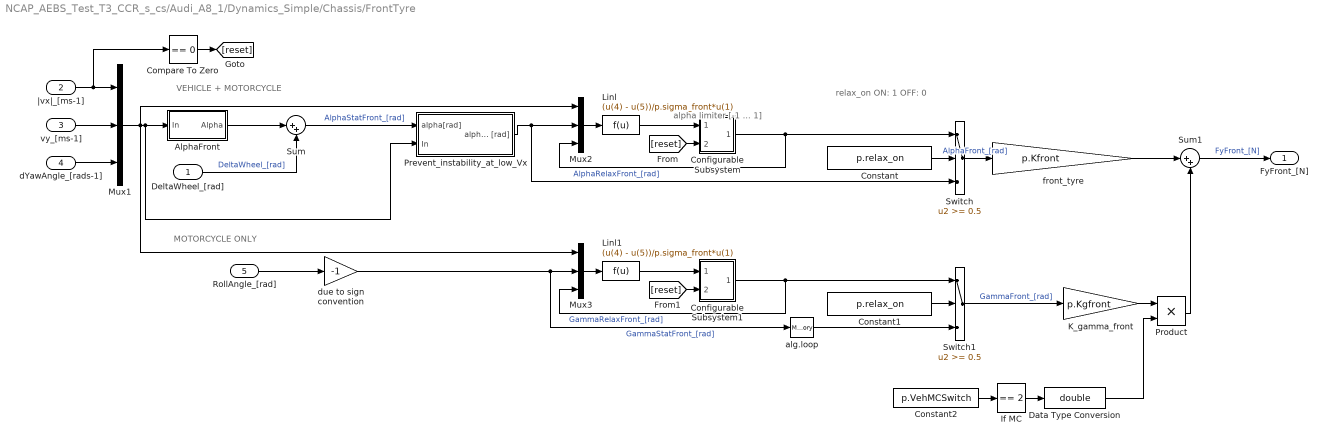
== system NCAP_AEBS_Test_T3_CCR_s_cs/Audi_A8_1/Dynamics_Simple/Chassis/FrontTyre ==
  note: alpha limiter
      | [-1 ... 1]
  note: relax_on
      | ON: 1
      | OFF: 0
  note: MOTORCYCLE ONLY
  note: VEHICLE + MOTORCYCLE
  DeltaWheel_[rad] : Inport
  |vx|_[ms-1] : Inport  Port=2
  vy_[ms-1] : Inport  Port=3
  dYawAngle_[rads-1] : Inport  Port=4
  RollAngle_[rad] : Inport  Port=5
  AlphaFront : Subsystem
  Compare To Zero : simulink/Logic and Bit Operations/Compare To Zero  SystemSampleTime=-1  relop===  LogicOutDataTypeMode=boolean  ZeroCross=off
  Configurable Subsystem : Subsystem  BlockChoice=Discrete-Time Integrator  mask{ComputationMode=ComputationMode}
      mask prompts: ComputationMode "Computation mode:"
      mask init:
      | SetComputationMode(gcb,ComputationMode);
      settings: AttributesFormatString=%<BlockChoice>  OpenFcn=BringToFront(gcb);  MemberBlocks=Discrete-Time Integrator,Integrator
      settings: TemplateBlock=|
      | PreScanSimulinkLibrary/Configurable Subsystems/integral with reset and limits
      | for slip angle/Configurable
      | Subsystem
  Configurable Subsystem1 : Subsystem  BlockChoice=Discrete-Time Integrator  mask{ComputationMode=ComputationMode}
      mask prompts: ComputationMode "Computation mode:"
      mask init:
      | SetComputationMode(gcb,ComputationMode);
      settings: AttributesFormatString=%<BlockChoice>  OpenFcn=BringToFront(gcb);  MemberBlocks=Discrete-Time Integrator,Integrator
      settings: TemplateBlock=|
      | PreScanSimulinkLibrary/Configurable Subsystems/integral with reset/Configurable
      | Subsystem
  Constant : Constant  Value=p.relax_on
  Constant1 : Constant  Value=p.relax_on
  Constant2 : Constant  Value=p.VehMCSwitch
  Data Type Conversion : DataTypeConversion  OutDataTypeStr=double
  If MC : simulink/Logic and Bit Operations/Compare To Constant  SystemSampleTime=-1  relop===  const=2  LogicOutDataTypeMode=uint8  ZeroCross=off
  K_gamma_front : Gain  Gain=p.Kgfront
  Linl : Fcn  Expr=(u(4) - u(5))/p.sigma_front*u(1)
  Linl1 : Fcn  Expr=(u(4) - u(5))/p.sigma_front*u(1)
  Mux1 : Mux  Inputs=3
  Mux2 : Mux  Inputs={3,1,1}
  Mux3 : Mux  Inputs={3,1,1}
  Prevent_instability_at_low_Vx : Subsystem
  Product : Product  RndMeth=Zero
  Sum : Sum  Inputs=|++  SaturateOnIntegerOverflow=on  InputSameDT=on  OutDataTypeStr=Inherit: Same as first input
  Sum1 : Sum  Inputs=|++
  Switch : Switch  Threshold=0.5  SaturateOnIntegerOverflow=on  InputSameDT=on
  Switch1 : Switch  Threshold=0.5  SaturateOnIntegerOverflow=on  InputSameDT=on
  alg.loop : Memory
  due to sign convention : Gain  Gain=-1  SaturateOnIntegerOverflow=on  OutDataTypeStr=Inherit: Same as input  ParamDataTypeStr=Inherit: Same as input
  front_tyre : Gain  Gain=p.Kfront
  FyFront_[N] : Outport
  wires:
  Prevent_instability_at_low_Vx/1(alpha [rad]) -> Mux2/2, Switch/3
  Sum/1 -> Prevent_instability_at_low_Vx/1(alpha[rad])  "AlphaStatFront_[rad]"
  Switch/1 -> front_tyre/1  "AlphaFront_[rad]"
  Constant/1 -> Switch/2
  Sum1/1 -> FyFront_[N]/1  "FyFront_[N]"
  Mux2/1 -> Linl/1
  Linl/1 -> Configurable Subsystem/1(In1)
  Configurable Subsystem/1(Out1) -> Mux2/3, Switch/1  "AlphaRelaxFront_[rad]"
  AlphaFront/1(Alpha) -> Sum/1
  Mux1/1 -> Prevent_instability_at_low_Vx/2(In), AlphaFront/1(In), Mux2/1, Mux3/1
  |vx|_[ms-1]/1 -> Mux1/1, Compare To Zero/1
  vy_[ms-1]/1 -> Mux1/2
  dYawAngle_[rads-1]/1 -> Mux1/3
  alg.loop/1 -> Switch1/3
  Configurable Subsystem1/1(Out1) -> Mux3/3, Switch1/1  "GammaRelaxFront_[rad]"
  Linl1/1 -> Configurable Subsystem1/1(In1)
  Mux3/1 -> Linl1/1
  Constant1/1 -> Switch1/2
  due to sign convention/1 -> alg.loop/1, Mux3/2  "GammaStatFront_[rad]"
  RollAngle_[rad]/1 -> due to sign convention/1
  front_tyre/1 -> Sum1/1
  Constant2/1 -> If MC/1
  If MC/1 -> Data Type Conversion/1
  K_gamma_front/1 -> Product/1
  Product/1 -> Sum1/2
  Data Type Conversion/1 -> Product/2
  Compare To Zero/1 -> [reset]
  [reset] -> Configurable Subsystem/2(In2)
  [reset] -> Configurable Subsystem1/2(In2)
  DeltaWheel_[rad]/1 -> Sum/2  "DeltaWheel_[rad]"
  Switch1/1 -> K_gamma_front/1  "GammaFront_[rad]"

== system NCAP_AEBS_Test_T3_CCR_s_cs/Audi_A8_1/Dynamics_Simple/Chassis/MuxDynState ==
  note: The position inputs are computed by the
      | integrated velocity.
  note: mode: Dynamics
      | VelVEHICLE
      | wrt VEH
  note: AnglesVEHICLE
      | wrtGLOB
  vx [ms-1] : Inport
  vy [ms-1] : Inport  Port=2
  vz [ms-1] : Inport  Port=3
  R [rad] : Inport  Port=4
  P [rad] : Inport  Port=5
  Y [rad] : Inport  Port=6
  Configurable Subsystem1 : Subsystem  BlockChoice=Integrator  mask{ComputationMode=ComputationMode}
      mask prompts: ComputationMode "Computation mode:"
      mask init:
      | SetComputationMode(gcb,ComputationMode);
      settings: AttributesFormatString=%<BlockChoice>  OpenFcn=BringToFront(gcb);  MemberBlocks=Discrete-Time Integrator,Integrator
      settings: TemplateBlock=|
      | PreScanSimulinkLibrary/Configurable Subsystems/integral/Configurable
      | Subsystem1
  Ground : Ground
  Ground1 : Ground
  Mux : Mux  Inputs=[3 3 3]
  Mux1 : Mux  Inputs=3
  Mux2 : Mux  Inputs=3
  Transformation_BODY2GLOBAL : Subsystem
  mux3 : Mux  Inputs=3
  State : Outport
  wires:
  Ground1/1 -> mux3/2  "pitch"
  Y [rad]/1 -> Mux2/3, mux3/3  "yaw"
  P [rad]/1 -> Mux2/2
  R [rad]/1 -> Mux2/1
  vz [ms-1]/1 -> Mux1/3
  vy [ms-1]/1 -> Mux1/2
  vx [ms-1]/1 -> Mux1/1
  Mux2/1 -> Mux/3
  Transformation_BODY2GLOBAL/1(Vvector_GLOBAL_[m/s]) -> Configurable Subsystem1/1(In1), Mux/2  "VelVEH wrt  GLOB"
  mux3/1 -> Transformation_BODY2GLOBAL/2(angles_BODYwrtGLOB_[rad])
  Ground/1 -> mux3/1  "roll"
  Mux/1 -> State/1
  Mux1/1 -> Transformation_BODY2GLOBAL/1(Vvector_BODY_[m/s])
  Configurable Subsystem1/1(Out1) -> Mux/1  "PosVEH wrt  GLOB"

== system NCAP_AEBS_Test_T3_CCR_s_cs/Audi_A8_1/Dynamics_Simple/Chassis/Power Assisted Steering ==
  note: MOTORCYCLE
  note: VEHICLE
  note: Reverse steering direction for negative velocities
  Vx_[ms-1] : Inport
  Delta_in_[deg] : Inport  Port=2
  Constant : Constant
  Constant1 : Constant  Value=p.VehMCSwitch
  Lookup Table : Lookup  InputValues=[0 35 45 100]  Table=[1 1 0.2 0.2]
  Multiport Switch : MultiPortSwitch  Inputs=2  zeroidx=off
  Product : Product  Inputs=3  RndMeth=Zero
  Sign : Signum
  Delta_out_[deg] : Outport
  wires:
  Vx_[ms-1]/1 -> Lookup Table/1, Sign/1
  Delta_in_[deg]/1 -> Product/3
  Constant1/1 -> Multiport Switch/1
  Constant/1 -> Multiport Switch/3
  Lookup Table/1 -> Multiport Switch/2
  Multiport Switch/1 -> Product/2
  Product/1 -> Delta_out_[deg]/1
  Sign/1 -> Product/1

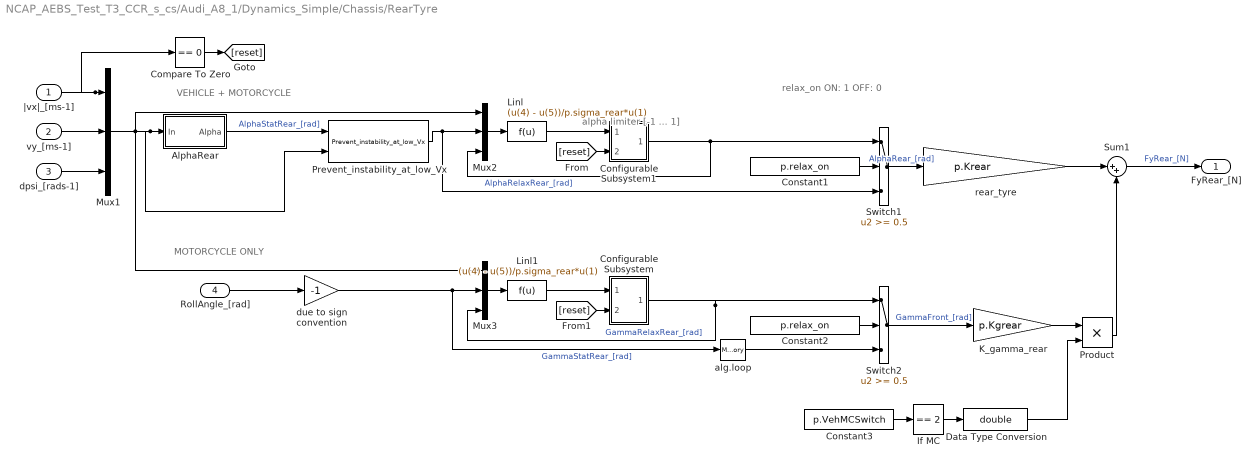
== system NCAP_AEBS_Test_T3_CCR_s_cs/Audi_A8_1/Dynamics_Simple/Chassis/RearTyre ==
  note: alpha limiter
      | [-1 ... 1]
  note: relax_on
      | ON: 1
      | OFF: 0
  note: MOTORCYCLE ONLY
  note: VEHICLE + MOTORCYCLE
  |vx|_[ms-1] : Inport
  vy_[ms-1] : Inport  Port=2
  dpsi_[rads-1] : Inport  Port=3
  RollAngle_[rad] : Inport  Port=4
  AlphaRear : Subsystem
  Compare To Zero : simulink/Logic and Bit Operations/Compare To Zero  SystemSampleTime=-1  relop===  LogicOutDataTypeMode=boolean  ZeroCross=off
  Configurable Subsystem : Subsystem  BlockChoice=Discrete-Time Integrator  mask{ComputationMode=ComputationMode}
      mask prompts: ComputationMode "Computation mode:"
      mask init:
      | SetComputationMode(gcb,ComputationMode);
      settings: AttributesFormatString=%<BlockChoice>  OpenFcn=BringToFront(gcb);  MemberBlocks=Discrete-Time Integrator,Integrator
      settings: TemplateBlock=|
      | PreScanSimulinkLibrary/Configurable Subsystems/integral with reset/Configurable
      | Subsystem
  Configurable Subsystem1 : Subsystem  BlockChoice=Discrete-Time Integrator  mask{ComputationMode=ComputationMode}
      mask prompts: ComputationMode "Computation mode:"
      mask init:
      | SetComputationMode(gcb,ComputationMode);
      settings: AttributesFormatString=%<BlockChoice>  OpenFcn=BringToFront(gcb);  MemberBlocks=Discrete-Time Integrator,Integrator
      settings: TemplateBlock=|
      | PreScanSimulinkLibrary/Configurable Subsystems/integral with reset and limits
      | for slip angle/Configurable
      | Subsystem
  Constant1 : Constant  Value=p.relax_on
  Constant2 : Constant  Value=p.relax_on
  Constant3 : Constant  Value=p.VehMCSwitch
  Data Type Conversion : DataTypeConversion  OutDataTypeStr=double
  If MC : simulink/Logic and Bit Operations/Compare To Constant  SystemSampleTime=-1  relop===  const=2  LogicOutDataTypeMode=uint8  ZeroCross=off
  K_gamma_rear : Gain  Gain=p.Kgrear
  Linl : Fcn  Expr=(u(4) - u(5))/p.sigma_rear*u(1)
  Linl1 : Fcn  Expr=(u(4) - u(5))/p.sigma_rear*u(1)
  Mux1 : Mux  Inputs=3
  Mux2 : Mux  Inputs={3,1,1}
  Mux3 : Mux  Inputs={3,1,1}
  Prevent_instability_at_low_Vx : PreScanSimulinkLibrary/Simple_Vehicle_Dynamics/Chassis/FrontTyre/Prevent_instability_at_low_Vx  SystemSampleTime=-1
  Product : Product  RndMeth=Zero
  Sum1 : Sum  Inputs=|++
  Switch1 : Switch  Threshold=0.5  SaturateOnIntegerOverflow=on  InputSameDT=on
  Switch2 : Switch  Threshold=0.5  SaturateOnIntegerOverflow=on  InputSameDT=on
  alg.loop : Memory
  due to sign convention : Gain  Gain=-1  SaturateOnIntegerOverflow=on  OutDataTypeStr=Inherit: Same as input  ParamDataTypeStr=Inherit: Same as input
  rear_tyre : Gain  Gain=p.Krear
  FyRear_[N] : Outport
  wires:
  Prevent_instability_at_low_Vx/1 -> Switch1/3, Mux2/2
  AlphaRear/1(Alpha) -> Prevent_instability_at_low_Vx/1  "AlphaStatRear_[rad]"
  Switch1/1 -> rear_tyre/1  "AlphaRear_[rad]"
  Constant1/1 -> Switch1/2
  Sum1/1 -> FyRear_[N]/1  "FyRear_[N]"
  Mux2/1 -> Linl/1
  Linl/1 -> Configurable Subsystem1/1(In1)
  Configurable Subsystem1/1(Out1) -> Mux2/3, Switch1/1  "AlphaRelaxRear_[rad]"
  Mux1/1 -> Prevent_instability_at_low_Vx/2, AlphaRear/1(In), Mux2/1, Mux3/1
  |vx|_[ms-1]/1 -> Mux1/1, Compare To Zero/1
  vy_[ms-1]/1 -> Mux1/2
  dpsi_[rads-1]/1 -> Mux1/3
  alg.loop/1 -> Switch2/3
  Configurable Subsystem/1(Out1) -> Mux3/3, Switch2/1  "GammaRelaxRear_[rad]"
  Linl1/1 -> Configurable Subsystem/1(In1)
  Mux3/1 -> Linl1/1
  Constant2/1 -> Switch2/2
  due to sign convention/1 -> alg.loop/1, Mux3/2  "GammaStatRear_[rad]"
  RollAngle_[rad]/1 -> due to sign convention/1
  Constant3/1 -> If MC/1
  If MC/1 -> Data Type Conversion/1
  Product/1 -> Sum1/2
  Data Type Conversion/1 -> Product/2
  K_gamma_rear/1 -> Product/1
  rear_tyre/1 -> Sum1/1
  Compare To Zero/1 -> [reset]
  [reset] -> Configurable Subsystem1/2(In2)
  [reset] -> Configurable Subsystem/2(In2)
  Switch2/1 -> K_gamma_rear/1  "GammaFront_[rad]"

== system NCAP_AEBS_Test_T3_CCR_s_cs/Audi_A8_1/Dynamics_Simple/Engine/Configurable Subsystem ==
  In1 : Inport
  Discrete Rate Limiter : DiscreteTransferFcn  Numerator="[  1-exp(-( (TimeStep) / 0.1) )  ]"  Denominator="[  1   -exp(-( (TimeStep) / 0.1) )   ]"  SampleTime=TimeStep
  Out1 : Outport
  wires:
  Discrete Rate Limiter/1 -> Out1/1
  In1/1 -> Discrete Rate Limiter/1

== system NCAP_AEBS_Test_T3_CCR_s_cs/Audi_A8_1/Dynamics_Simple/Engine/Configurable Subsystem1 ==
  In1 : Inport
  Discrete-Time Integrator : DiscreteIntegrator  InitialCondition=p.rot_ini  SampleTime=TimeStep  LimitOutput=on  UpperSaturationLimit=p.rot_upp  LowerSaturationLimit=p.rot_low  ICPrevOutput=DiscIntNeverNeededParam  ICPrevScaledInput=DiscIntNeverNeededParam
  Out1 : Outport
  wires:
  Discrete-Time Integrator/1 -> Out1/1
  In1/1 -> Discrete-Time Integrator/1

== system NCAP_AEBS_Test_T3_CCR_s_cs/Audi_A8_1/Dynamics_Simple/Gear: Auto Manual/If Action Subsystem ==
  In1 : Inport
  Action Port : ActionPort  PropagateVarSize=During execution
  Out1 : Outport
  wires:
  In1/1 -> Out1/1

== system NCAP_AEBS_Test_T3_CCR_s_cs/Audi_A8_1/Dynamics_Simple/Gear: Auto Manual/If Action Subsystem1 ==
  In1 : Inport
  Action Port : ActionPort  PropagateVarSize=During execution
  Out1 : Outport
  wires:
  In1/1 -> Out1/1

== system NCAP_AEBS_Test_T3_CCR_s_cs/Audi_A8_1/Dynamics_Simple/ShiftLogic/Detect Increase ==
  GearNr_[-] : Inport
  In2 : Inport  Port=2
  Constant : Constant
  Data Type Conversion : DataTypeConversion  OutDataTypeStr=double
  Data Type Conversion1 : DataTypeConversion  OutDataTypeStr=double
  Detect Increase : simulink/Logic and Bit Operations/Detect Increase  SystemSampleTime=-1  vinit=1
  If : If  NumInputs=2  IfExpression="u1==1 &  u2==1"
  If V0 higher of the from 2->3 shifting velocity : Subsystem  TreatAsAtomicUnit=on
  Merge : Merge
  Other : Subsystem  TreatAsAtomicUnit=on
  Out1 : Outport
  wires:
  If/2 -> Other/Action
  If V0 higher of the from 2->3 shifting velocity/1(Out1) -> Merge/1
  Other/1(Out1) -> Merge/2
  Detect Increase/1 -> Data Type Conversion/1
  Merge/1 -> Out1/1
  If/1 -> If V0 higher of the from 2->3 shifting velocity/Action
  Data Type Conversion1/1 -> If/2
  Data Type Conversion/1 -> If/1
  Constant/1 -> If V0 higher of the from 2->3 shifting velocity/1(In1)
  GearNr_[-]/1 -> Detect Increase/1
  In2/1 -> Data Type Conversion1/1, Other/1(In1)

== system NCAP_AEBS_Test_T3_CCR_s_cs/Audi_A8_1/Dynamics_Simple/ShiftLogic/If Action Neutral ==
  In1 : Inport
  Action Port : ActionPort  InitializeStates=reset  PropagateVarSize=During execution
  Out1 : Outport
  wires:
  In1/1 -> Out1/1

== system NCAP_AEBS_Test_T3_CCR_s_cs/Audi_A8_1/Dynamics_Simple/ShiftLogic/If Action Normal ==
  In1 : Inport
  Action Port : ActionPort  InitializeStates=reset  PropagateVarSize=During execution
  Out1 : Outport
  wires:
  In1/1 -> Out1/1

== system NCAP_AEBS_Test_T3_CCR_s_cs/Audi_A8_1/Dynamics_Simple/ShiftLogic/If Action Reverse ==
  In1 : Inport
  Action Port : ActionPort  InitializeStates=reset  PropagateVarSize=During execution
  Out1 : Outport
  wires:
  In1/1 -> Out1/1

== system NCAP_AEBS_Test_T3_CCR_s_cs/Audi_A8_1/Dynamics_Simple/Transmission/Torque_Converter ==
  note: To compensate for no hydraulic connection when in neutral gear
  note: > 0
  note: <= 0
  nEngine_[rpm] : Inport
  nTransmission_[rpm] : Inport  Port=2
  Gear nr : Inport  Port=3
  Compare To Constant : simulink/Logic and Bit Operations/Compare To Constant  SystemSampleTime=-1  relop=<=  const=1  LogicOutDataTypeMode=uint8  ZeroCross=off
  Compare To Zero : simulink/Logic and Bit Operations/Compare To Zero  SystemSampleTime=-1  relop=~=  LogicOutDataTypeMode=uint8  ZeroCross=off
  Constant : Constant  Value=1/50
  Constant1 : Constant
  Constant2 : Constant
  Drag : Gain  Gain=-1
  FactorK : Lookup  InputValues=p.speedratio  Table=p.Kfactor*p.Kcorr  SaturateOnIntegerOverflow=on
  Impeller : Fcn  Expr=u^2
  Product : Product  RndMeth=Zero
  Product1 : Product  RndMeth=Zero
  Quotient : Product  Inputs=*/  SaturateOnIntegerOverflow=on  InputSameDT=on  OutDataTypeStr=Inherit: Same as first input
  SpeedRatio : Product  Inputs=*/  SaturateOnIntegerOverflow=on  InputSameDT=on  OutDataTypeStr=Inherit: Same as first input
  Sum : Sum  Inputs=|+-
  Switch : Switch  Criteria=u2 ~= 0  Threshold=0.5
  Switch1 : Switch  Criteria=u2 ~= 0
  TorqueRatio : Lookup  InputValues=[p.speedratio 1]  Table=[p.Torqueratio 0]  SaturateOnIntegerOverflow=on
  Turbine : Product  SaturateOnIntegerOverflow=on  InputSameDT=on  OutDataTypeStr=Inherit: Same as first input
  ImpellerTorque_[Nm] : Outport  InitialOutput=0
  TurbineTorque_[Nm] : Outport  Port=2  InitialOutput=0
  wires:
  nTransmission_[rpm]/1 -> SpeedRatio/1
  nEngine_[rpm]/1 -> Quotient/1, SpeedRatio/2
  Impeller/1 -> Product/2, Turbine/1
  SpeedRatio/1 -> FactorK/1, TorqueRatio/1, Compare To Constant/1, Sum/1
  FactorK/1 -> Quotient/2
  Quotient/1 -> Impeller/1
  Product/1 -> ImpellerTorque_[Nm]/1
  Switch/1 -> Product/1, Product1/1
  Constant/1 -> Switch/3
  Constant1/1 -> Switch/1
  Gear nr/1 -> Compare To Zero/1
  Compare To Zero/1 -> Switch/2
  Switch1/1 -> Product1/2
  Product1/1 -> TurbineTorque_[Nm]/1
  Drag/1 -> Switch1/3
  Sum/1 -> Drag/1
  Constant2/1 -> Sum/2
  Compare To Constant/1 -> Switch1/2
  TorqueRatio/1 -> Turbine/2
  Turbine/1 -> Switch1/1

== system NCAP_AEBS_Test_T3_CCR_s_cs/Audi_A8_1/Dynamics_Simple/Transmission/Transmission_Ratio ==
  tTransmissionIn_[Nm] : Inport
  GearNr_[-] : Inport  Port=2
  nTransmissionOut_[rpm] : Inport  Port=3
  Ensure positive TransmissionRPM : Abs
  If : If  IfExpression=u1 == 0  ElseIfExpressions=u1 == -1
  If Action Neutral : Subsystem  TreatAsAtomicUnit=on
  If Action Normal : Subsystem  TreatAsAtomicUnit=on
  If Action Reverse : Subsystem  TreatAsAtomicUnit=on
  Merge : Merge  Inputs=3
  OutputTorque = 0 : Constant  Value=0
  Product : Product  SaturateOnIntegerOverflow=on  InputSameDT=on  OutDataTypeStr=Inherit: Same as first input
  Product1 : Product  SaturateOnIntegerOverflow=on  InputSameDT=on  OutDataTypeStr=Inherit: Same as first input
  Transmission Gear ratios : Lookup  InputValues=p.tr_in  Table=p.tr_out  SaturateOnIntegerOverflow=on
  tTransmissionOut_[Nm] : Outport  InitialOutput=0
  nTransmissionIn_[rpm] : Outport  Port=2  InitialOutput=0
  wires:
  GearNr_[-]/1 -> Transmission Gear ratios/1, If/1
  If/3 -> If Action Normal/Action
  If/2 -> If Action Reverse/Action
  If Action Normal/1(Out1) -> Merge/3
  If Action Reverse/1(Out1) -> Merge/2
  If/1 -> If Action Neutral/Action
  If Action Neutral/1(Out1) -> Merge/1
  Product1/1 -> Ensure positive TransmissionRPM/1
  Merge/1 -> tTransmissionOut_[Nm]/1
  Product/1 -> If Action Reverse/1(In1), If Action Normal/1(In1)
  OutputTorque = 0/1 -> If Action Neutral/1(In1)
  Transmission Gear ratios/1 -> Product/2, Product1/1
  nTransmissionOut_[rpm]/1 -> Product1/2
  tTransmissionIn_[Nm]/1 -> Product/1
  Ensure positive TransmissionRPM/1 -> nTransmissionIn_[rpm]/1

== system NCAP_AEBS_Test_T3_CCR_s_cs/Audi_A8_1/PathFollower_1/CTRL REFERENCES/Calculate Preview Point (pvp) by extrapolating current Vehicle Position (p0) with Preview Distance and Vehicle Orientation ==
  Preview Distance : Inport
  x,y,Y Demux [m,m,rad] : Inport  Port=2
  Demux : Demux  Outputs=3
  Fcn : Fcn  Expr=u(2)*cos(u(1))
  Fcn1 : Fcn  Expr=u(2)*sin(u(1))
  Mux : Mux  Inputs=2
  Sum : Sum  Inputs=|++
  Sum1 : Sum  Inputs=|++
  x_glob_PVD : Outport
  y_glob_PVD : Outport  Port=2
  Y [rad] : Outport  Port=3
  wires:
  Demux/3 -> Mux/1, Y [rad]/1
  Demux/1 -> Sum/1
  Demux/2 -> Sum1/1
  Preview Distance/1 -> Mux/2
  Mux/1 -> Fcn/1, Fcn1/1
  Fcn/1 -> Sum/2
  Fcn1/1 -> Sum1/2
  Sum/1 -> x_glob_PVD/1
  Sum1/1 -> y_glob_PVD/1
  x,y,Y Demux [m,m,rad]/1 -> Demux/1

== system NCAP_AEBS_Test_T3_CCR_s_cs/Audi_A8_1/PathFollower_1/DELTA CTRL/Error check ==
  Add3 : Sum  Inputs=-+
  Demux : Demux  Outputs=2
  Selector1 : Selector  InputPortWidth=3  IndexOptions=Index vector (dialog)  Indices=[1 2]  OutputSizes=1
  p0_x error : Scope
      settings: YMin=-0.2  YMax=0.2
  p0_y error : Scope
      settings: YMin=-0.2  YMax=0.2  SaveName=ScopeData2
  wires:
  Demux/2 -> p0_y error/1
  Add3/1 -> Demux/1
  Demux/1 -> p0_x error/1
  [pref0] -> Add3/2
  [p0] -> Selector1/1
  Selector1/1 -> Add3/1

== system NCAP_AEBS_Test_T3_CCR_s_cs/Audi_A8_1/PathFollower_1/THROTTLE CTRL/If Desired Velocity = 0 ==
  In1 : Inport
  Action Port : ActionPort  InitializeStates=reset  PropagateVarSize=During execution
  constant : Constant  Value=0
  constant1 : Constant  Value=150
  throttle [%] : Outport  InitialOutput=[0]
  brake pressure [bar] : Outport  Port=2  InitialOutput=[150]
  Auto_GearShift : Outport  Port=3
  wires:
  constant1/1 -> brake pressure [bar]/1
  constant/1 -> throttle [%]/1
  In1/1 -> Auto_GearShift/1

== system NCAP_AEBS_Test_T3_CCR_s_cs/Audi_A8_1/PathFollower_1/THROTTLE CTRL/If Desired Velocity ~= 0 ==
  note: CONSTANT VELOCITY CONTROL
  note: No brake/throttle actions
      | in case of small ctrl error,
      |  in order to prevent nervous
      | ctrl behaviour
  In1 : Inport
  Desired Velocity [m/s] : Inport  Port=2
  Action Port : ActionPort  InitializeStates=reset  PropagateVarSize=During execution
  Dead Zone : DeadZone  LowerValue=-10  UpperValue=1  SaturateOnIntegerOverflow=on
  Gain11 : Gain  Gain=10
  Gain6 : Gain  Gain=-1
  Limiter_brake : Saturate  UpperLimit=150  LowerLimit=0
  Limiter_throttle : Saturate  UpperLimit=100  LowerLimit=0
  PID Controller : simulink_need_slupdate/PID Controller  SystemSampleTime=-1  P=20  I=0.3  D=3.065
  throttle [%] : Outport
  brake pressure [bar] : Outport  Port=2
  Auto_GearShift : Outport  Port=3
  wires:
  Limiter_throttle/1 -> throttle [%]/1  "throttle"
  Limiter_brake/1 -> brake pressure [bar]/1
  Gain6/1 -> Limiter_brake/1
  Gain11/1 -> Gain6/1
  Dead Zone/1 -> Limiter_throttle/1, Gain11/1
  Desired Velocity [m/s]/1 -> PID Controller/1
  PID Controller/1 -> Dead Zone/1
  In1/1 -> Auto_GearShift/1
